simulink model "Powertrain_model_HEV"  (R2021a)
settings: Solver=VariableStepAuto  StartTime=0.0  StopTime=10.0  RelTol=1e-3
values from neighbouring files (symbols this model uses):
  DR = 5.213    [Sim_script.m]    (also in workspace.mat)
  eta_EM_map = [0.5831 0.6831 0.781 0.826 0 0 0 0 0 0.6107 0.7107 0.8049 ... (270 elements, 9x30)]    [workspace.mat]
  MaxLimit = [2.1951    294.39 ... (first row only)    [power_distribute_func.m]
  P_CE_idle = 0    [Sim_script.m]    (also in workspace.mat = 1)
  T_EM_col = [-74.73 -59.49 -53.55 -49.77 -44.93 -40 -34.96 -30.36 -25.1 -20.31 -15.68 -10.18 ... (30 elements, 30x1)]    [workspace.mat]
  T_EM_max = [70 70 70 52 38 28 19 13 9]    [workspace.mat]
  Trans_In = 24.086    [Sim_script.m]    (also in workspace.mat)
  w_CE_idle = 400    [Sim_script.m]    (also in workspace.mat = 32)
  w_EM_row = [0 75 150 225 300 375 450 525 600]    [workspace.mat]
undefined symbols (not defined in the file or in its folder): dailyloadl, eta_EG_map, Res_Torque, T_EG_max, w_EG_row, w_EG_upper
libraries: visionstatistics x1, pid_lib x1
settings Model: Creator=user  LastModifiedBy=user

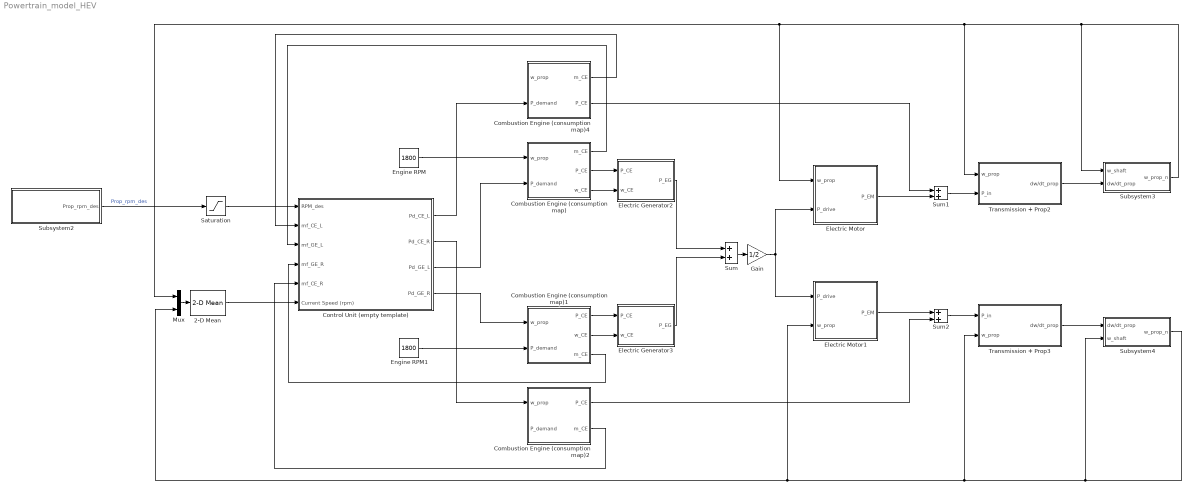
== system Powertrain_model_HEV ==
  2-D Mean : visionstatistics/2-D Mean  run=off  reset_popup=None  directionMode=Entire input  dimension=1  treatSBRowAsCol=on  outputLastDataTypeStr=Inherit: Same as accumulator  accumMode=Binary point scaling  accumWordLength=32  accumFracLength=0  accumLastDataTypeStr=fixdt([],32,0)  roiEnable=off  roiType=Rectangles  roiPortion=Entire ROI  roiOutput=Individual statistics for each ROI  roiFlag=off  roundingMode=Floor  overflowMode=off  accumDataTypeStr=fixdt([],32,0)  outputDataTypeStr=Inherit: Same as accumulator  outputMin=[]  outputMax=[]
      settings: SourceProductBaseCode=VP
  Combustion Engine (consumption map) : Subsystem  Tag=combustion engine  AncestorBlock=|
      | qss_tb_library/Energy Converter/Combustion Engine
      | (consumption map)
  Combustion Engine (consumption map)1 : Subsystem  Tag=combustion engine  AncestorBlock=|
      | qss_tb_library/Energy Converter/Combustion Engine
      | (consumption map)
  Combustion Engine (consumption map)2 : Subsystem  Tag=combustion engine  AncestorBlock=|
      | qss_tb_library/Energy Converter/Combustion Engine
      | (consumption map)
  Combustion Engine (consumption map)4 : Subsystem  Tag=combustion engine  AncestorBlock=|
      | qss_tb_library/Energy Converter/Combustion Engine
      | (consumption map)
  Control Unit (empty template) : Subsystem  Tag=control unit  AncestorBlock=|
      | qss_tb_library/Controller/Control Unit
      | (empty template)
  Electric Generator2 : Subsystem  AncestorBlock=qss_tb_library/Energy Converter/Electric Generator
  Electric Generator3 : Subsystem  AncestorBlock=qss_tb_library/Energy Converter/Electric Generator
  Electric Motor : Subsystem  AncestorBlock=qss_tb_library/Energy Converter/Electric Motor
  Electric Motor1 : Subsystem  AncestorBlock=qss_tb_library/Energy Converter/Electric Motor  mask(Electric Motor){emmapname='qss_em_original_map', scale_EM=1, theta_EM=0.1, P_aux=0}
      mask prompts: emmapname "Motor map name"; scale_EM "Motor scaling factor [-]"; theta_EM "Motor inertia [kg*m2]"; P_aux "Power required by auxiliaries [W]"
      mask help:
      | This block simulates the behaviour of an electric motor. The block is based on an efficiency map. The map is located in the Data/EnergyConvertter/ElectricMotor directory.
      |
      | Input:
      | =====
      | 	w_gear		Speed of the fly wheel [rad/s]
      | 	dw_gear	Acceleration of the fly wheel [rad/s^2]
      | 	T_gear		Torque on the fly wheel [Nm]
      |
      | Output:
      | ======
      | 	P_EM		Power produced by the electric motor [W]
      |
      | Motor map:
      | ======
      | The motor map file must contain the following variables:
      | eta_EM_map		% Efficiency map                [-]
      | w_EM_row		% Motor speed range             [rad/s]
      | T_EM_col		% Motor torque range            [Nm]
      | w_EM_max		% Maximum motor speed           [rad/s]
      | load T_EM_max	% Maximum motor torque          [Nm]
      mask init:
      | init_EM;
  Engine RPM : Constant  Value=1800
  Engine RPM1 : Constant  Value=1800
  Gain : Gain  Gain=1/2
  Mux : Mux  Inputs=2
  Saturation : Saturate  UpperLimit=inf  LowerLimit=w_CE_idle
  Subsystem2 : Subsystem  TreatAsAtomicUnit=on
  Subsystem3 : Subsystem
  Subsystem4 : Subsystem
  Sum : Sum
  Sum1 : Sum
  Sum2 : Sum
  Transmission + Prop2 : Subsystem
  Transmission + Prop3 : Subsystem
  wires:
  Combustion Engine (consumption map)1/1(P_CE) -> Electric Generator3/1(P_CE)
  Engine RPM/1 -> Combustion Engine (consumption map)/1(w_prop)
  Combustion Engine (consumption map)/2(P_CE) -> Electric Generator2/1(P_CE)
  Transmission + Prop2/1(dw/dt_prop) -> Subsystem3/2(dw/dt_prop)
  Transmission + Prop3/1(dw/dt_prop) -> Subsystem4/1(dw/dt_prop)
  Subsystem3/1(w_prop_n) -> Subsystem3/1(w_shaft), Transmission + Prop2/1(w_prop), Electric Motor/1(w_prop), Mux/1
  Electric Motor1/1(P_EM) -> Sum2/1
  Combustion Engine (consumption map)1/2(w_CE) -> Electric Generator3/2(w_CE)
  Subsystem4/1(w_prop_n) -> Subsystem4/2(w_shaft), Transmission + Prop3/2(w_prop), Mux/2, Electric Motor1/2(w_prop)
  Electric Generator3/1(P_EG) -> Sum/2
  Sum2/1 -> Transmission + Prop3/1(P_in)
  Combustion Engine (consumption map)4/2(P_CE) -> Sum1/1
  Sum1/1 -> Transmission + Prop2/2(P_in)
  Gain/1 -> Electric Motor/2(P_drive), Electric Motor1/1(P_drive)
  Combustion Engine (consumption map)/1(m_CE) -> Control Unit (empty template)/3(mf_GE_L)
  Electric Motor/1(P_EM) -> Sum1/2
  Control Unit (empty template)/4(Pd_GE_R) -> Combustion Engine (consumption map)1/1(w_prop)
  Combustion Engine (consumption map)/3(w_CE) -> Electric Generator2/2(w_CE)
  Combustion Engine (consumption map)2/2(m_CE) -> Control Unit (empty template)/5(mf_CE_R)
  Combustion Engine (consumption map)4/1(m_CE) -> Control Unit (empty template)/2(mf_CE_L)
  Engine RPM1/1 -> Combustion Engine (consumption map)1/2(P_demand)
  Electric Generator2/1(P_EG) -> Sum/1
  Mux/1 -> 2-D Mean/1
  Control Unit (empty template)/3(Pd_GE_L) -> Combustion Engine (consumption map)/2(P_demand)
  Control Unit (empty template)/2(Pd_CE_R) -> Combustion Engine (consumption map)2/1(w_prop)
  Sum/1 -> Gain/1
  Control Unit (empty template)/1(Pd_CE_L) -> Combustion Engine (consumption map)4/2(P_demand)
  2-D Mean/1 -> Control Unit (empty template)/6(Current Speed (rpm))
  Combustion Engine (consumption map)1/3(m_CE) -> Control Unit (empty template)/4(mf_GE_R)
  Combustion Engine (consumption map)2/1(P_CE) -> Sum2/2
  Subsystem2/1(Prop_rpm_des) -> Saturation/1  "Prop_rpm_des"
  Saturation/1 -> Control Unit (empty template)/1(RPM_des)

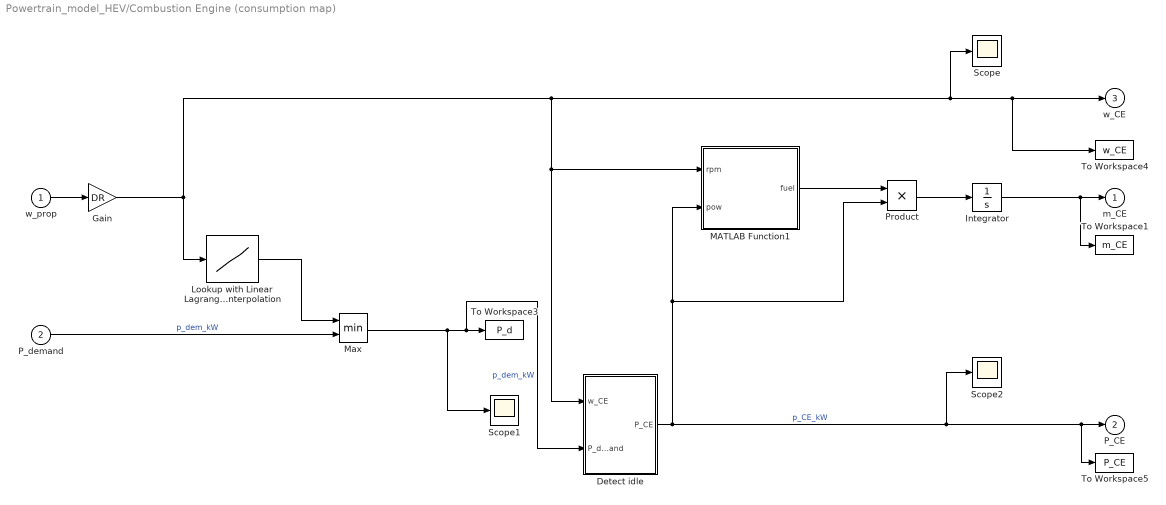
== system Powertrain_model_HEV/Combustion Engine (consumption map) ==
  w_prop : Inport
  P_demand : Inport  Port=2
  Detect idle : Subsystem
  Gain : Gain  Gain=DR
  Integrator : Integrator
  Lookup with Linear Lagrange Interpolation : Lookup_n-D  NumberOfTableDimensions=1  BreakpointsForDimension1=MaxLimit.('RPM')  Table=MaxLimit.('Pow_kW_')  InterpMethod=Linear Lagrange  InternalRulePriority=Speed  RndMeth=Simplest  InputSameDT=on
  MATLAB Function1 : MATLAB Function  TreatAsAtomicUnit=on
  Max : MinMax  Inputs=2
  Product : Product
  Scope : Scope
  Scope1 : Scope
  Scope2 : Scope
  To Workspace1 : ToWorkspace  VariableName=m_CE  SampleTime=-1
      settings: Save2DSignal=2-D array (concatenate along first dimension)
  To Workspace3 : ToWorkspace  VariableName=P_d  SampleTime=-1
      settings: Save2DSignal=2-D array (concatenate along first dimension)
  To Workspace4 : ToWorkspace  VariableName=w_CE  SampleTime=-1
      settings: Save2DSignal=2-D array (concatenate along first dimension)
  To Workspace5 : ToWorkspace  VariableName=P_CE  SampleTime=-1
      settings: Save2DSignal=2-D array (concatenate along first dimension)
  m_CE : Outport  InitialOutput=0
  P_CE : Outport  Port=2  InitialOutput=0
  w_CE : Outport  Port=3  InitialOutput=0
  wires:
  Integrator/1 -> To Workspace1/1, m_CE/1
  w_prop/1 -> Gain/1
  Detect idle/1(P_CE) -> Scope2/1, To Workspace5/1, P_CE/1, Product/2, MATLAB Function1/2(pow)  "p_CE_kW"
  Lookup with Linear Lagrange Interpolation/1 -> Max/1
  MATLAB Function1/1(fuel) -> Product/1
  Gain/1 -> w_CE/1, To Workspace4/1, Scope/1, Detect idle/1(w_CE), MATLAB Function1/1(rpm), Lookup with Linear Lagrange Interpolation/1
  Product/1 -> Integrator/1
  Max/1 -> Scope1/1, Detect idle/2(P_demand), To Workspace3/1  "p_dem_kW"
  P_demand/1 -> Max/2  "p_dem_kW"

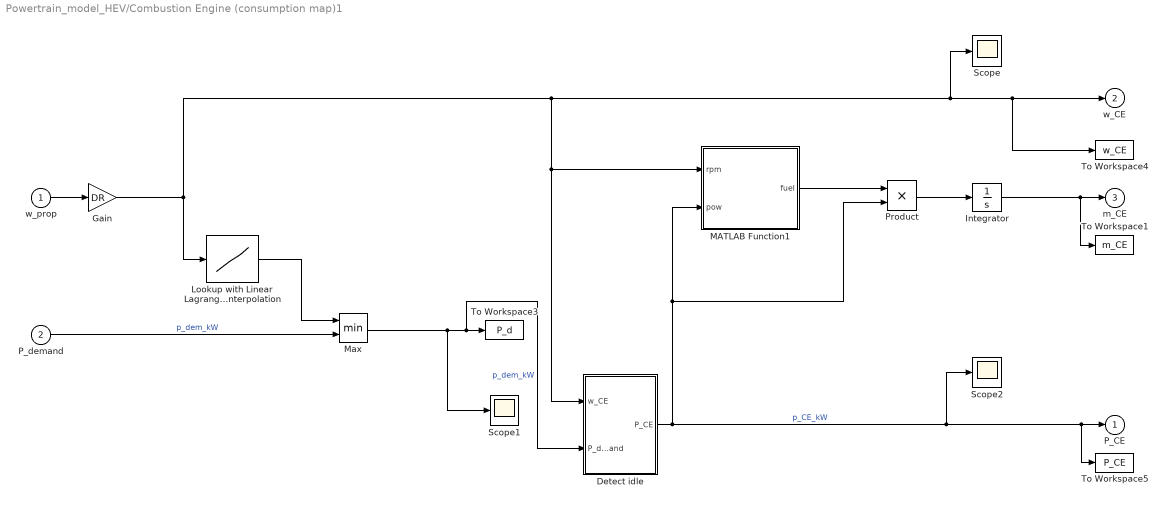
== system Powertrain_model_HEV/Combustion Engine (consumption map)1 ==
  w_prop : Inport
  P_demand : Inport  Port=2
  Detect idle : Subsystem
  Gain : Gain  Gain=DR
  Integrator : Integrator
  Lookup with Linear Lagrange Interpolation : Lookup_n-D  NumberOfTableDimensions=1  BreakpointsForDimension1=MaxLimit.('RPM')  Table=MaxLimit.('Pow_kW_')  InterpMethod=Linear Lagrange  InternalRulePriority=Speed  RndMeth=Simplest  InputSameDT=on
  MATLAB Function1 : MATLAB Function  TreatAsAtomicUnit=on
  Max : MinMax  Inputs=2
  Product : Product
  Scope : Scope
  Scope1 : Scope
  Scope2 : Scope
  To Workspace1 : ToWorkspace  VariableName=m_CE  SampleTime=-1
      settings: Save2DSignal=2-D array (concatenate along first dimension)
  To Workspace3 : ToWorkspace  VariableName=P_d  SampleTime=-1
      settings: Save2DSignal=2-D array (concatenate along first dimension)
  To Workspace4 : ToWorkspace  VariableName=w_CE  SampleTime=-1
      settings: Save2DSignal=2-D array (concatenate along first dimension)
  To Workspace5 : ToWorkspace  VariableName=P_CE  SampleTime=-1
      settings: Save2DSignal=2-D array (concatenate along first dimension)
  P_CE : Outport  InitialOutput=0
  w_CE : Outport  Port=2  InitialOutput=0
  m_CE : Outport  Port=3  InitialOutput=0
  wires:
  Integrator/1 -> To Workspace1/1, m_CE/1
  w_prop/1 -> Gain/1
  Detect idle/1(P_CE) -> Scope2/1, To Workspace5/1, P_CE/1, Product/2, MATLAB Function1/2(pow)  "p_CE_kW"
  Lookup with Linear Lagrange Interpolation/1 -> Max/1
  MATLAB Function1/1(fuel) -> Product/1
  Gain/1 -> w_CE/1, To Workspace4/1, Scope/1, Detect idle/1(w_CE), MATLAB Function1/1(rpm), Lookup with Linear Lagrange Interpolation/1
  Product/1 -> Integrator/1
  Max/1 -> Scope1/1, Detect idle/2(P_demand), To Workspace3/1  "p_dem_kW"
  P_demand/1 -> Max/2  "p_dem_kW"

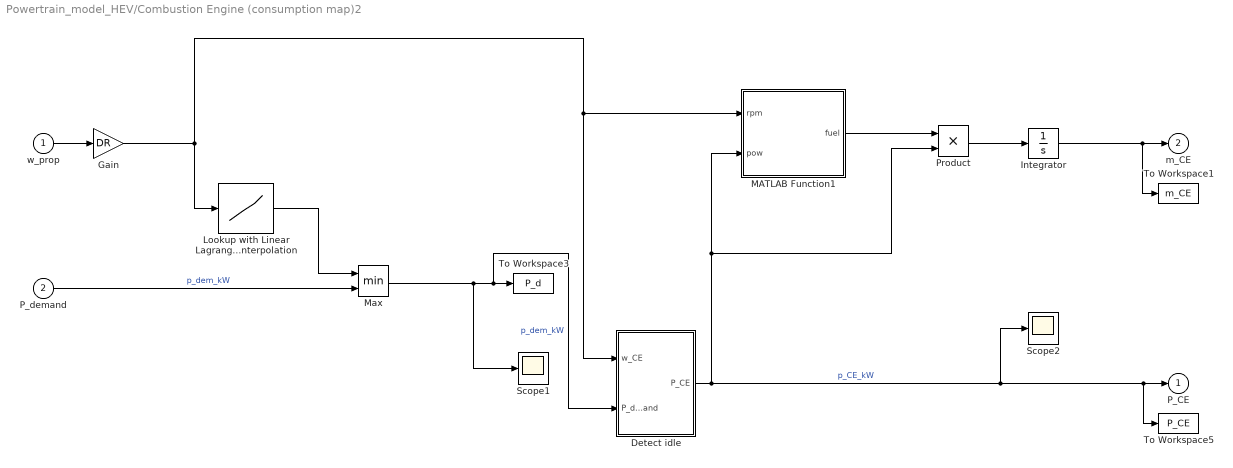
== system Powertrain_model_HEV/Combustion Engine (consumption map)2 ==
  w_prop : Inport
  P_demand : Inport  Port=2
  Detect idle : Subsystem
  Gain : Gain  Gain=DR
  Integrator : Integrator
  Lookup with Linear Lagrange Interpolation : Lookup_n-D  NumberOfTableDimensions=1  BreakpointsForDimension1=MaxLimit.('RPM')  Table=MaxLimit.('Pow_kW_')  InterpMethod=Linear Lagrange  InternalRulePriority=Speed  RndMeth=Simplest  InputSameDT=on
  MATLAB Function1 : MATLAB Function  TreatAsAtomicUnit=on
  Max : MinMax  Inputs=2
  Product : Product
  Scope1 : Scope
  Scope2 : Scope
  To Workspace1 : ToWorkspace  VariableName=m_CE  SampleTime=-1
      settings: Save2DSignal=2-D array (concatenate along first dimension)
  To Workspace3 : ToWorkspace  VariableName=P_d  SampleTime=-1
      settings: Save2DSignal=2-D array (concatenate along first dimension)
  To Workspace5 : ToWorkspace  VariableName=P_CE  SampleTime=-1
      settings: Save2DSignal=2-D array (concatenate along first dimension)
  P_CE : Outport  InitialOutput=0
  m_CE : Outport  Port=2  InitialOutput=0
  wires:
  Integrator/1 -> To Workspace1/1, m_CE/1
  w_prop/1 -> Gain/1
  Detect idle/1(P_CE) -> Scope2/1, To Workspace5/1, P_CE/1, Product/2, MATLAB Function1/2(pow)  "p_CE_kW"
  Lookup with Linear Lagrange Interpolation/1 -> Max/1
  MATLAB Function1/1(fuel) -> Product/1
  Gain/1 -> Detect idle/1(w_CE), MATLAB Function1/1(rpm), Lookup with Linear Lagrange Interpolation/1
  Product/1 -> Integrator/1
  Max/1 -> Scope1/1, Detect idle/2(P_demand), To Workspace3/1  "p_dem_kW"
  P_demand/1 -> Max/2  "p_dem_kW"

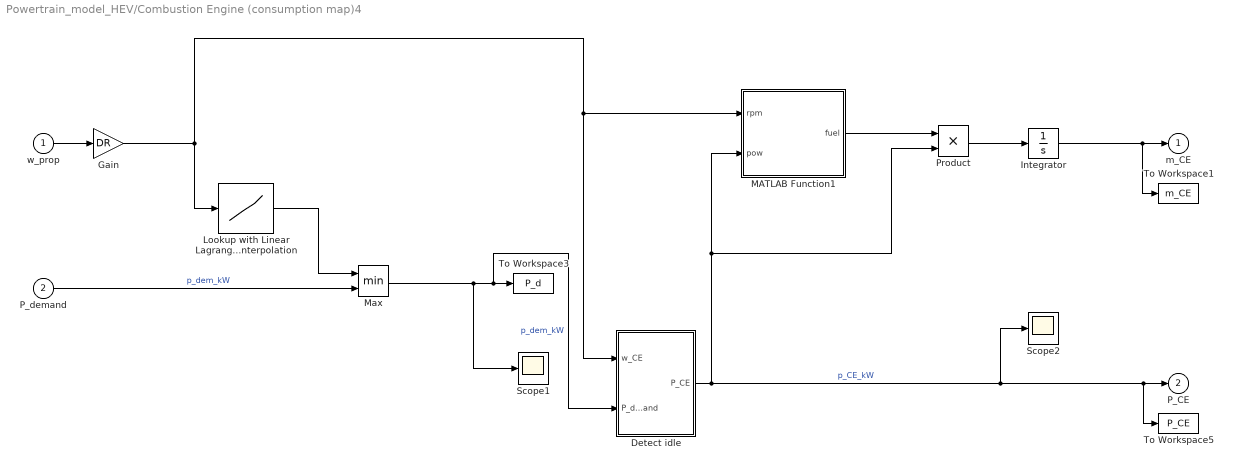
== system Powertrain_model_HEV/Combustion Engine (consumption map)4 ==
  w_prop : Inport
  P_demand : Inport  Port=2
  Detect idle : Subsystem
  Gain : Gain  Gain=DR
  Integrator : Integrator
  Lookup with Linear Lagrange Interpolation : Lookup_n-D  NumberOfTableDimensions=1  BreakpointsForDimension1=MaxLimit.('RPM')  Table=MaxLimit.('Pow_kW_')  InterpMethod=Linear Lagrange  InternalRulePriority=Speed  RndMeth=Simplest  InputSameDT=on
  MATLAB Function1 : MATLAB Function  TreatAsAtomicUnit=on
  Max : MinMax  Inputs=2
  Product : Product
  Scope1 : Scope
  Scope2 : Scope
  To Workspace1 : ToWorkspace  VariableName=m_CE  SampleTime=-1
      settings: Save2DSignal=2-D array (concatenate along first dimension)
  To Workspace3 : ToWorkspace  VariableName=P_d  SampleTime=-1
      settings: Save2DSignal=2-D array (concatenate along first dimension)
  To Workspace5 : ToWorkspace  VariableName=P_CE  SampleTime=-1
      settings: Save2DSignal=2-D array (concatenate along first dimension)
  m_CE : Outport  InitialOutput=0
  P_CE : Outport  Port=2  InitialOutput=0
  wires:
  Integrator/1 -> To Workspace1/1, m_CE/1
  w_prop/1 -> Gain/1
  Detect idle/1(P_CE) -> Scope2/1, To Workspace5/1, P_CE/1, Product/2, MATLAB Function1/2(pow)  "p_CE_kW"
  Lookup with Linear Lagrange Interpolation/1 -> Max/1
  MATLAB Function1/1(fuel) -> Product/1
  Gain/1 -> Detect idle/1(w_CE), MATLAB Function1/1(rpm), Lookup with Linear Lagrange Interpolation/1
  Product/1 -> Integrator/1
  Max/1 -> Scope1/1, Detect idle/2(P_demand), To Workspace3/1  "p_dem_kW"
  P_demand/1 -> Max/2  "p_dem_kW"

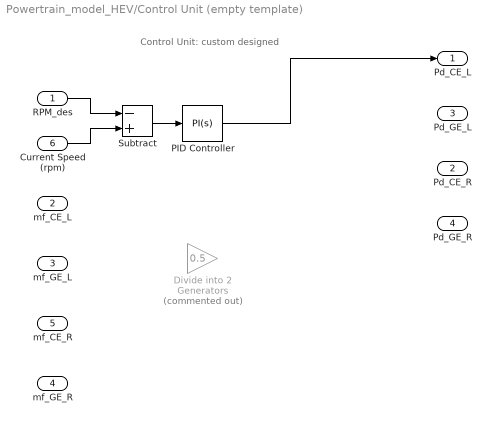
== system Powertrain_model_HEV/Control Unit (empty template) ==
  note: Control Unit: custom designed
  RPM_des : Inport
  mf_CE_L : Inport  Port=2
  mf_GE_L : Inport  Port=3
  mf_GE_R : Inport  Port=4
  mf_CE_R : Inport  Port=5
  Current Speed (rpm) : Inport  Port=6
  Divide into 2 Generators : Gain  Commented=on  Gain=0.5
  PID Controller : pid_lib/PID Controller  Controller=PI  Form=Parallel  TimeDomain=Continuous-time  UseExternalTs=off  SampleTime=-1  IntegratorMethod=Forward Euler  FilterMethod=Forward Euler  ControllerParametersSource=internal  P=4  I=1.2  D=0  UseFilter=on  N=100  TunerSelectOption=Transfer Function Based (PID Tuner App)  InitialConditionSource=internal  InitialConditionForIntegrator=0  InitialConditionForFilter=0  DifferentiatorICPrevScaledInput=0  ExternalReset=none  TrackingMode=off  Kt=1  LimitOutput=off  SatLimitsSource=internal  UpperSaturationLimit=inf  LowerSaturationLimit=-inf  LinearizeAsGain=on  AntiWindupMode=none  Kb=1  POutMin=[]  POutMax=[]  IOutMin=[]  IOutMax=[]  DOutMin=[]  DOutMax=[]  NOutMin=[]  NOutMax=[]  SumOutMin=[]  SumOutMax=[]  SaturationOutMin=[]  SaturationOutMax=[]  PParamMin=[]  PParamMax=[]  IParamMin=[]  IParamMax=[]  DParamMin=[]  DParamMax=[]  NParamMin=[]  NParamMax=[]  KbParamMin=[]  KbParamMax=[]  KtParamMin=[]  KtParamMax=[]  KbOutMin=[]  KbOutMax=[]  KtOutMin=[]  KtOutMax=[]  IntegratorOutMin=[]  IntegratorOutMax=[]  FilterOutMin=[]  FilterOutMax=[]  SumI1OutMin=[]  SumI1OutMax=[]  SumI2OutMin=[]  SumI2OutMax=[]  SumI3OutMin=[]  SumI3OutMax=[]  SumI4OutMin=[]  SumI4OutMax=[]  SumDOutMin=[]  SumDOutMax=[]  DifferentiatorOutMin=[]  DifferentiatorOutMax=[]  FilterDiffOutCoefMin=[]  FilterDiffOutCoefMax=[]  ReciprocalOutMin=[]  ReciprocalOutMax=[]  SumDenOutMin=[]  SumDenOutMax=[]  SumNumOutMin=[]  SumNumOutMax=[]  DivideOutMin=[]  DivideOutMax=[]  UdiffTsProdOutMin=[]  UdiffTsProdOutMax=[]  NTsProdOutMin=[]  NTsProdOutMax=[]  UintegralTsProdOutMin=[]  UintegralTsProdOutMax=[]  UngainTsProdOutMin=[]  UngainTsProdOutMax=[]  IntegratorContinuousStateAttributes=''  IntegratorStateMustResolveToSignalObject=off  IntegratorRTWStateStorageClass=Auto  FilterContinuousStateAttributes=''  FilterStateMustResolveToSignalObject=off  FilterRTWStateStorageClass=Auto  ParallelPVariant=InternalParameters  IdealPVariant=Disabled  IVariant=InternalParameters  DVariant=Disabled  IntegratorVariant=Continuous  SatVariant=Disabled  AWVariant=Passthrough  PCopyVariant=Disabled  TRVariant=Disabled  FdbkBlocksVariant=Forward  IdealPFdbkVariant=Disabled  SatFdbkVariant=Disabled  DerivativeFilterVariant=Disabled  NVariant=Disabled  NCopyVariant=Disabled_SignalSpec  FilterICVariant=Disabled  IntegratorICVariant=InternalICs  ExternalResetVariant=Disabled  TRSumVariant=Passthrough  SumFdbkVariant=Disabled  SumVariant=Sum_PI  TsampFilterVariant=InternalTs  TsampNgainVariant=Passthrough  TsampIntegralVariant=Passthrough  ExternalSaturationOutDataTypeStr=Inherit: Same as second input
  Subtract : Sum  Inputs=-+
  Pd_CE_L : Outport  InitialOutput=0
  Pd_CE_R : Outport  Port=2  InitialOutput=0
  Pd_GE_L : Outport  Port=3  InitialOutput=0
  Pd_GE_R : Outport  Port=4  InitialOutput=0
  wires:
  Current Speed (rpm)/1 -> Subtract/2
  RPM_des/1 -> Subtract/1
  PID Controller/1 -> Pd_CE_L/1
  Subtract/1 -> PID Controller/1

== system Powertrain_model_HEV/Electric Generator2 ==
  P_CE : Inport
  w_CE : Inport  Port=2
  Detect overload and overspeed : Subsystem
  Divide : Product  Inputs=/*
  "Efficiency eta = f(w, T)" : Lookup2D  RowIndex=w_EG_row  ColumnIndex=T_EG_col  Table=eta_EG_map
  Product : Product  Inputs=3  InputSameDT=on  RndMeth=Zero  SaturateOnIntegerOverflow=on  OutDataTypeStr=Inherit: Same as first input
  To Workspace1 : ToWorkspace  VariableName=w_EG  SampleTime=-1
  To Workspace2 : ToWorkspace  VariableName=T_EG  SampleTime=-1
  To Workspace5 : ToWorkspace  VariableName=P_EG  SampleTime=-1
  P_EG : Outport  InitialOutput=0
  wires:
  Product/1 -> To Workspace5/1, P_EG/1
  "Efficiency eta = f(w, T)"/1 -> Product/1
  Divide/1 -> To Workspace2/1, Detect overload and overspeed/2(T_EG), "Efficiency eta = f(w, T)"/2, Product/2
  P_CE/1 -> Divide/2
  w_CE/1 -> To Workspace1/1, Detect overload and overspeed/1(w_EG), "Efficiency eta = f(w, T)"/1, Product/3, Divide/1

== system Powertrain_model_HEV/Electric Generator3 ==
  P_CE : Inport
  w_CE : Inport  Port=2
  Detect overload and overspeed : Subsystem
  Divide : Product  Inputs=/*
  "Efficiency eta = f(w, T)" : Lookup2D  RowIndex=w_EG_row  ColumnIndex=T_EG_col  Table=eta_EG_map
  Product : Product  Inputs=3  InputSameDT=on  RndMeth=Zero  SaturateOnIntegerOverflow=on  OutDataTypeStr=Inherit: Same as first input
  To Workspace1 : ToWorkspace  VariableName=w_EG  SampleTime=-1
  To Workspace2 : ToWorkspace  VariableName=T_EG  SampleTime=-1
  To Workspace5 : ToWorkspace  VariableName=P_EG  SampleTime=-1
  P_EG : Outport  InitialOutput=0
  wires:
  Product/1 -> To Workspace5/1, P_EG/1
  "Efficiency eta = f(w, T)"/1 -> Product/1
  Divide/1 -> To Workspace2/1, Detect overload and overspeed/2(T_EG), "Efficiency eta = f(w, T)"/2, Product/2
  P_CE/1 -> Divide/2
  w_CE/1 -> To Workspace1/1, Detect overload and overspeed/1(w_EG), "Efficiency eta = f(w, T)"/1, Product/3, Divide/1

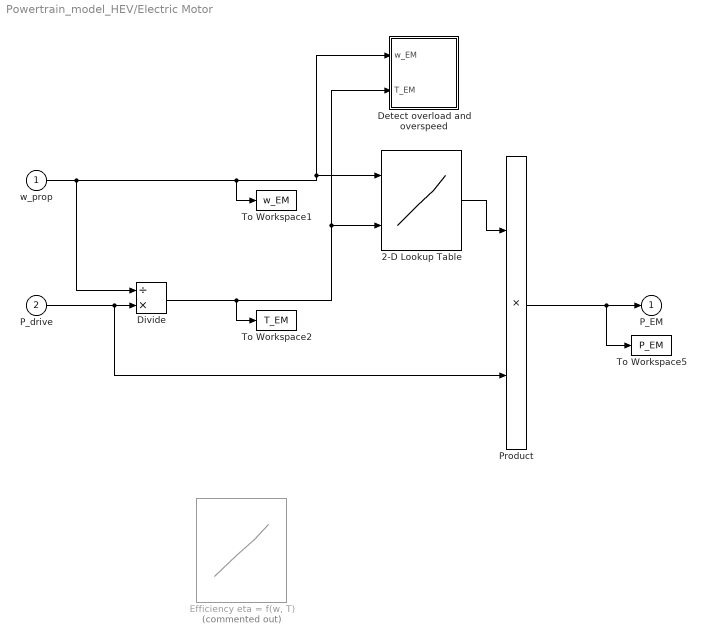
== system Powertrain_model_HEV/Electric Motor ==
  w_prop : Inport
  P_drive : Inport  Port=2
  2-D Lookup Table : Lookup_n-D  BreakpointsForDimension1=w_EM_row  BreakpointsForDimension2=T_EM_col  Table=eta_EM_map  InterpMethod=Cubic spline  ExtrapMethod=Cubic spline  InternalRulePriority=Speed  RndMeth=Simplest  InputSameDT=on
      settings: InputPortMap=u0,u1
  Detect overload and overspeed : Subsystem
  Divide : Product  Inputs=/*
  "Efficiency eta = f(w, T)" : Lookup2D  Commented=on  RowIndex=w_EM_row  ColumnIndex=T_EM_col  Table=eta_EM_map
  Product : Product  InputSameDT=on  RndMeth=Zero  SaturateOnIntegerOverflow=on  OutDataTypeStr=Inherit: Same as first input
  To Workspace1 : ToWorkspace  VariableName=w_EM  SampleTime=-1
  To Workspace2 : ToWorkspace  VariableName=T_EM  SampleTime=-1
  To Workspace5 : ToWorkspace  VariableName=P_EM  SampleTime=-1
  P_EM : Outport  InitialOutput=0
  wires:
  Product/1 -> To Workspace5/1, P_EM/1
  Divide/1 -> To Workspace2/1, 2-D Lookup Table/2, Detect overload and overspeed/2(T_EM)
  P_drive/1 -> Product/2, Divide/2
  2-D Lookup Table/1 -> Product/1
  w_prop/1 -> Divide/1, To Workspace1/1, 2-D Lookup Table/1, Detect overload and overspeed/1(w_EM)

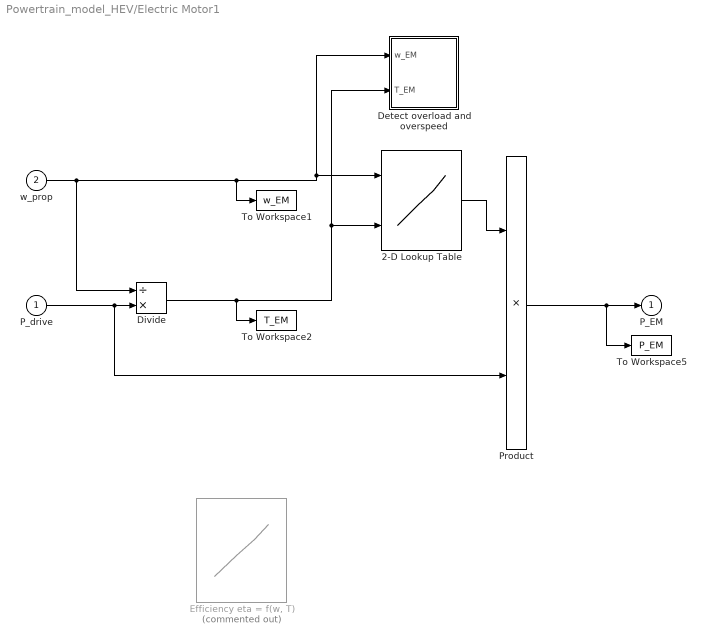
== system Powertrain_model_HEV/Electric Motor1 ==
  P_drive : Inport
  w_prop : Inport  Port=2
  2-D Lookup Table : Lookup_n-D  BreakpointsForDimension1=w_EM_row  BreakpointsForDimension2=T_EM_col  Table=eta_EM_map  InterpMethod=Cubic spline  ExtrapMethod=Cubic spline  InternalRulePriority=Speed  RndMeth=Simplest  InputSameDT=on
      settings: InputPortMap=u0,u1
  Detect overload and overspeed : Subsystem
  Divide : Product  Inputs=/*
  "Efficiency eta = f(w, T)" : Lookup2D  Commented=on  RowIndex=w_EM_row  ColumnIndex=T_EM_col  Table=eta_EM_map
  Product : Product  InputSameDT=on  RndMeth=Zero  SaturateOnIntegerOverflow=on  OutDataTypeStr=Inherit: Same as first input
  To Workspace1 : ToWorkspace  VariableName=w_EM  SampleTime=-1
  To Workspace2 : ToWorkspace  VariableName=T_EM  SampleTime=-1
  To Workspace5 : ToWorkspace  VariableName=P_EM  SampleTime=-1
  P_EM : Outport  InitialOutput=0
  wires:
  w_prop/1 -> Detect overload and overspeed/1(w_EM), 2-D Lookup Table/1, To Workspace1/1, Divide/1
  2-D Lookup Table/1 -> Product/1
  P_drive/1 -> Divide/2, Product/2
  Divide/1 -> Detect overload and overspeed/2(T_EM), 2-D Lookup Table/2, To Workspace2/1
  Product/1 -> P_EM/1, To Workspace5/1

== system Powertrain_model_HEV/Subsystem2 ==
  1-D Lookup Table : Lookup_n-D  NumberOfTableDimensions=1  BreakpointsForDimension1=[1:10800]  Table=dailyloadl.('m_sec')  InternalRulePriority=Speed  RndMeth=Simplest  InputSameDT=on
  Clock : Clock
  To Workspace3 : ToWorkspace  VariableName=t  SampleTime=-1
      settings: Save2DSignal=2-D array (concatenate along first dimension)
  To Workspace4 : ToWorkspace  VariableName=rpm_des  SampleTime=-1
      settings: Save2DSignal=2-D array (concatenate along first dimension)
  Prop_rpm_des : Outport
  wires:
  Clock/1 -> To Workspace3/1, 1-D Lookup Table/1
  1-D Lookup Table/1 -> Prop_rpm_des/1, To Workspace4/1

== system Powertrain_model_HEV/Subsystem3 ==
  w_shaft : Inport
  dw/dt_prop : Inport  Port=2
  Add : Sum
  Gain : Gain  Gain=1/9.5493
  Gain1 : Gain  Gain=1/DR
  Integrator : Integrator  InitialCondition=w_CE_idle
  Saturation : Saturate  UpperLimit=inf  LowerLimit=w_CE_idle
  w_prop_n : Outport
  wires:
  dw/dt_prop/1 -> Integrator/1
  Integrator/1 -> Gain/1
  Saturation/1 -> w_prop_n/1
  Gain/1 -> Add/2
  w_shaft/1 -> Gain1/1
  Gain1/1 -> Add/1
  Add/1 -> Saturation/1

== system Powertrain_model_HEV/Subsystem4 ==
  dw/dt_prop : Inport
  w_shaft : Inport  Port=2
  Add : Sum
  Gain : Gain  Gain=1/9.5493
  Gain1 : Gain  Gain=1/DR
  Integrator : Integrator  InitialCondition=w_CE_idle
  Saturation : Saturate  UpperLimit=inf  LowerLimit=w_CE_idle
  w_prop_n : Outport
  wires:
  dw/dt_prop/1 -> Integrator/1
  Integrator/1 -> Gain/1
  Saturation/1 -> w_prop_n/1
  Gain/1 -> Add/2
  w_shaft/1 -> Gain1/1
  Gain1/1 -> Add/1
  Add/1 -> Saturation/1

== system Powertrain_model_HEV/Transmission + Prop2 ==
  w_prop : Inport
  P_in : Inport  Port=2
  Divide : Product  Inputs=*/
  Drive Ratio : Gain  Gain=DR
  Gain : Gain  Gain=DR
  Gain2 : Gain  Gain=9.5488*1000
  Gearbox+Prop Inertia : Gain  Gain=1/Trans_In
  Lookup with Linear Point-slope Interpolation : Lookup_n-D  NumberOfTableDimensions=1  BreakpointsForDimension1=Res_Torque.('RPMEngine')  Table=Res_Torque.('TorqueNM')  InternalRulePriority=Speed  RndMeth=Simplest  InputSameDT=on
  Scope : Scope
  Subtract : Sum  Inputs=+-
  dw/dt_prop : Outport
  wires:
  Lookup with Linear Point-slope Interpolation/1 -> Subtract/2  "T_res"
  P_in/1 -> Divide/1
  Subtract/1 -> Scope/1, Drive Ratio/1
  Gearbox+Prop Inertia/1 -> dw/dt_prop/1  "dw/dt_prop"
  Drive Ratio/1 -> Gearbox+Prop Inertia/1
  Divide/1 -> Gain2/1  "T_CE"
  Gain/1 -> Divide/2, Lookup with Linear Point-slope Interpolation/1
  Gain2/1 -> Subtract/1
  w_prop/1 -> Gain/1  "prop_rads"

== system Powertrain_model_HEV/Transmission + Prop3 ==
  P_in : Inport
  w_prop : Inport  Port=2
  Divide : Product  Inputs=*/
  Drive Ratio : Gain  Gain=DR
  Gain : Gain  Gain=DR
  Gain2 : Gain  Gain=9.5488*1000
  Gearbox+Prop Inertia : Gain  Gain=1/Trans_In
  Lookup with Linear Point-slope Interpolation : Lookup_n-D  NumberOfTableDimensions=1  BreakpointsForDimension1=Res_Torque.('RPMEngine')  Table=Res_Torque.('TorqueNM')  InternalRulePriority=Speed  RndMeth=Simplest  InputSameDT=on
  Scope : Scope
  Subtract : Sum  Inputs=+-
  dw/dt_prop : Outport
  wires:
  Lookup with Linear Point-slope Interpolation/1 -> Subtract/2  "T_res"
  P_in/1 -> Divide/1
  Subtract/1 -> Scope/1, Drive Ratio/1
  Gearbox+Prop Inertia/1 -> dw/dt_prop/1  "dw/dt_prop"
  Drive Ratio/1 -> Gearbox+Prop Inertia/1
  Divide/1 -> Gain2/1  "T_CE"
  Gain/1 -> Divide/2, Lookup with Linear Point-slope Interpolation/1
  Gain2/1 -> Subtract/1
  w_prop/1 -> Gain/1  "prop_rads"

== system Powertrain_model_HEV/Combustion Engine (consumption map)/Detect idle ==
  w_CE : Inport
  P_demand : Inport  Port=2
  Constant3 : Constant  Value=P_CE_idle
  Idle detection : Fcn  Expr=(u(1) <= w_CE_idle) * (u(2) <= P_CE_idle)
  Mux : Mux  Inputs=2
  P_demand1 : InportShadow  Port=2
  Switch2 : Switch  Threshold=0.5  SaturateOnIntegerOverflow=on  InputSameDT=on
  P_CE : Outport  InitialOutput=0
  wires:
  Constant3/1 -> Switch2/1
  Switch2/1 -> P_CE/1
  P_demand1/1 -> Switch2/3
  Idle detection/1 -> Switch2/2
  w_CE/1 -> Mux/1
  P_demand/1 -> Mux/2
  Mux/1 -> Idle detection/1

== system Powertrain_model_HEV/Combustion Engine (consumption map)1/Detect idle ==
  w_CE : Inport
  P_demand : Inport  Port=2
  Constant3 : Constant  Value=P_CE_idle
  Idle detection : Fcn  Expr=(u(1) <= w_CE_idle) * (u(2) <= P_CE_idle)
  Mux : Mux  Inputs=2
  P_demand1 : InportShadow  Port=2
  Switch2 : Switch  Threshold=0.5  SaturateOnIntegerOverflow=on  InputSameDT=on
  P_CE : Outport  InitialOutput=0
  wires:
  Constant3/1 -> Switch2/1
  Switch2/1 -> P_CE/1
  P_demand1/1 -> Switch2/3
  Idle detection/1 -> Switch2/2
  w_CE/1 -> Mux/1
  P_demand/1 -> Mux/2
  Mux/1 -> Idle detection/1

== system Powertrain_model_HEV/Combustion Engine (consumption map)2/Detect idle ==
  w_CE : Inport
  P_demand : Inport  Port=2
  Constant3 : Constant  Value=P_CE_idle
  Idle detection : Fcn  Expr=(u(1) <= w_CE_idle) * (u(2) <= P_CE_idle)
  Mux : Mux  Inputs=2
  P_demand1 : InportShadow  Port=2
  Switch2 : Switch  Threshold=0.5  SaturateOnIntegerOverflow=on  InputSameDT=on
  P_CE : Outport  InitialOutput=0
  wires:
  Constant3/1 -> Switch2/1
  Switch2/1 -> P_CE/1
  P_demand1/1 -> Switch2/3
  Idle detection/1 -> Switch2/2
  w_CE/1 -> Mux/1
  P_demand/1 -> Mux/2
  Mux/1 -> Idle detection/1

== system Powertrain_model_HEV/Combustion Engine (consumption map)4/Detect idle ==
  w_CE : Inport
  P_demand : Inport  Port=2
  Constant3 : Constant  Value=P_CE_idle
  Idle detection : Fcn  Expr=(u(1) <= w_CE_idle) * (u(2) <= P_CE_idle)
  Mux : Mux  Inputs=2
  P_demand1 : InportShadow  Port=2
  Switch2 : Switch  Threshold=0.5  SaturateOnIntegerOverflow=on  InputSameDT=on
  P_CE : Outport  InitialOutput=0
  wires:
  Constant3/1 -> Switch2/1
  Switch2/1 -> P_CE/1
  P_demand1/1 -> Switch2/3
  Idle detection/1 -> Switch2/2
  w_CE/1 -> Mux/1
  P_demand/1 -> Mux/2
  Mux/1 -> Idle detection/1

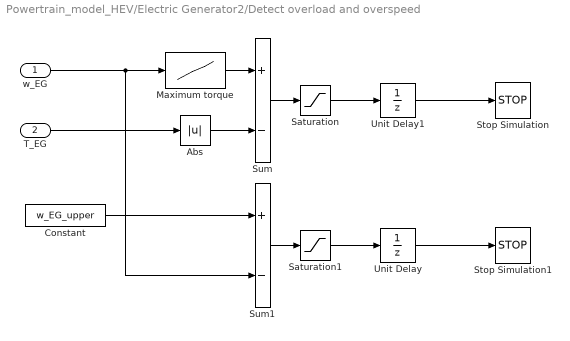
== system Powertrain_model_HEV/Electric Generator2/Detect overload and overspeed ==
  w_EG : Inport
  T_EG : Inport  Port=2
  Abs : Abs  SaturateOnIntegerOverflow=on
  Constant : Constant  Value=w_EG_upper
  Maximum torque : Lookup  InputValues=w_EG_row  Table=T_EG_max  SaturateOnIntegerOverflow=on
  Saturation : Saturate  UpperLimit=0  LowerLimit=-inf
  Saturation1 : Saturate  UpperLimit=0  LowerLimit=-inf
  Stop Simulation : Stop
  Stop Simulation1 : Stop
  Sum : Sum  Inputs=+-  InputSameDT=on  SaturateOnIntegerOverflow=on  OutDataTypeStr=Inherit: Same as first input
  Sum1 : Sum  Inputs=+-  InputSameDT=on  SaturateOnIntegerOverflow=on  OutDataTypeStr=Inherit: Same as first input
  Unit Delay : UnitDelay  SampleTime=-1  HasFrameUpgradeWarning=on
  Unit Delay1 : UnitDelay  SampleTime=-1  HasFrameUpgradeWarning=on
  wires:
  Unit Delay1/1 -> Stop Simulation/1
  Unit Delay/1 -> Stop Simulation1/1
  Saturation1/1 -> Unit Delay/1
  Sum1/1 -> Saturation1/1
  Constant/1 -> Sum1/1
  Saturation/1 -> Unit Delay1/1
  Abs/1 -> Sum/2
  Maximum torque/1 -> Sum/1
  T_EG/1 -> Abs/1
  w_EG/1 -> Sum1/2, Maximum torque/1
  Sum/1 -> Saturation/1

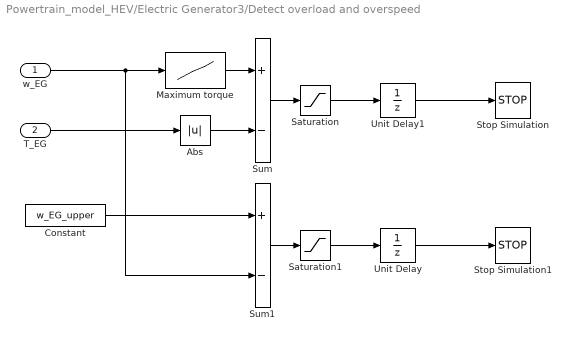
== system Powertrain_model_HEV/Electric Generator3/Detect overload and overspeed ==
  w_EG : Inport
  T_EG : Inport  Port=2
  Abs : Abs  SaturateOnIntegerOverflow=on
  Constant : Constant  Value=w_EG_upper
  Maximum torque : Lookup  InputValues=w_EG_row  Table=T_EG_max  SaturateOnIntegerOverflow=on
  Saturation : Saturate  UpperLimit=0  LowerLimit=-inf
  Saturation1 : Saturate  UpperLimit=0  LowerLimit=-inf
  Stop Simulation : Stop
  Stop Simulation1 : Stop
  Sum : Sum  Inputs=+-  InputSameDT=on  SaturateOnIntegerOverflow=on  OutDataTypeStr=Inherit: Same as first input
  Sum1 : Sum  Inputs=+-  InputSameDT=on  SaturateOnIntegerOverflow=on  OutDataTypeStr=Inherit: Same as first input
  Unit Delay : UnitDelay  SampleTime=-1  HasFrameUpgradeWarning=on
  Unit Delay1 : UnitDelay  SampleTime=-1  HasFrameUpgradeWarning=on
  wires:
  Unit Delay1/1 -> Stop Simulation/1
  Unit Delay/1 -> Stop Simulation1/1
  Saturation1/1 -> Unit Delay/1
  Sum1/1 -> Saturation1/1
  Constant/1 -> Sum1/1
  Saturation/1 -> Unit Delay1/1
  Abs/1 -> Sum/2
  Maximum torque/1 -> Sum/1
  T_EG/1 -> Abs/1
  w_EG/1 -> Sum1/2, Maximum torque/1
  Sum/1 -> Saturation/1

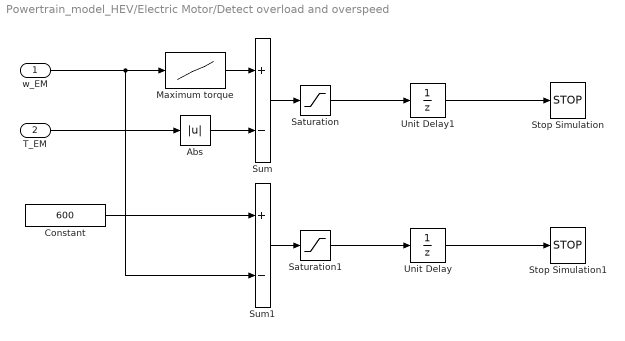
== system Powertrain_model_HEV/Electric Motor/Detect overload and overspeed ==
  w_EM : Inport
  T_EM : Inport  Port=2
  Abs : Abs  SaturateOnIntegerOverflow=on
  Constant : Constant  Value=600
  Maximum torque : Lookup  InputValues=w_EM_row  Table=T_EM_max  SaturateOnIntegerOverflow=on
  Saturation : Saturate  UpperLimit=0  LowerLimit=-inf
  Saturation1 : Saturate  UpperLimit=0  LowerLimit=-inf
  Stop Simulation : Stop
  Stop Simulation1 : Stop
  Sum : Sum  Inputs=+-  InputSameDT=on  SaturateOnIntegerOverflow=on  OutDataTypeStr=Inherit: Same as first input
  Sum1 : Sum  Inputs=+-  InputSameDT=on  SaturateOnIntegerOverflow=on  OutDataTypeStr=Inherit: Same as first input
  Unit Delay : UnitDelay  SampleTime=-1  HasFrameUpgradeWarning=on
  Unit Delay1 : UnitDelay  SampleTime=-1  HasFrameUpgradeWarning=on
  wires:
  Unit Delay1/1 -> Stop Simulation/1
  Unit Delay/1 -> Stop Simulation1/1
  Sum/1 -> Saturation/1
  w_EM/1 -> Maximum torque/1, Sum1/2
  T_EM/1 -> Abs/1
  Maximum torque/1 -> Sum/1
  Abs/1 -> Sum/2
  Saturation/1 -> Unit Delay1/1
  Constant/1 -> Sum1/1
  Sum1/1 -> Saturation1/1
  Saturation1/1 -> Unit Delay/1

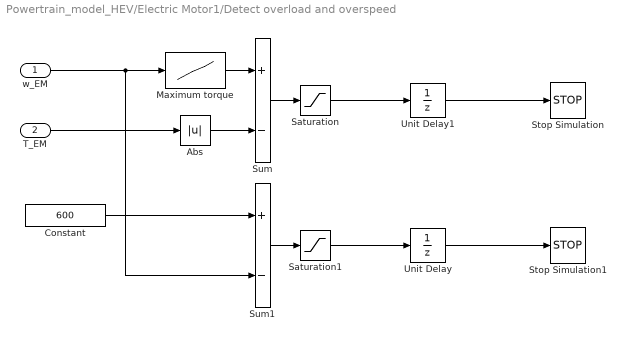
== system Powertrain_model_HEV/Electric Motor1/Detect overload and overspeed ==
  w_EM : Inport
  T_EM : Inport  Port=2
  Abs : Abs  SaturateOnIntegerOverflow=on
  Constant : Constant  Value=600
  Maximum torque : Lookup  InputValues=w_EM_row  Table=T_EM_max  SaturateOnIntegerOverflow=on
  Saturation : Saturate  UpperLimit=0  LowerLimit=-inf
  Saturation1 : Saturate  UpperLimit=0  LowerLimit=-inf
  Stop Simulation : Stop
  Stop Simulation1 : Stop
  Sum : Sum  Inputs=+-  InputSameDT=on  SaturateOnIntegerOverflow=on  OutDataTypeStr=Inherit: Same as first input
  Sum1 : Sum  Inputs=+-  InputSameDT=on  SaturateOnIntegerOverflow=on  OutDataTypeStr=Inherit: Same as first input
  Unit Delay : UnitDelay  SampleTime=-1  HasFrameUpgradeWarning=on
  Unit Delay1 : UnitDelay  SampleTime=-1  HasFrameUpgradeWarning=on
  wires:
  Saturation1/1 -> Unit Delay/1
  Sum1/1 -> Saturation1/1
  Constant/1 -> Sum1/1
  Saturation/1 -> Unit Delay1/1
  Abs/1 -> Sum/2
  Maximum torque/1 -> Sum/1
  T_EM/1 -> Abs/1
  w_EM/1 -> Sum1/2, Maximum torque/1
  Sum/1 -> Saturation/1
  Unit Delay/1 -> Stop Simulation1/1
  Unit Delay1/1 -> Stop Simulation/1

== matlab function Powertrain_model_HEV/Combustion Engine (consumption map)1/MATLAB Function1 ==
  data: rpm input; fuel output; pow input
function fuel   = fuel_con_map(rpm,pow)
x = (rpm-1180)/409.7;
y = (pow-876.1)/438.6;
p00 =         203;
p10 =      0.9394;
p01 =      -8.327;
p20 =       1.894;
p11 =     -0.7168;
p02 =       1.321;
p30 =      0.2621;
p21 =       1.482;
p12 =       5.529;
p03 =      -2.619;
p40 =      0.9252;
p31 =      -3.236;
p22 =       3.413;
p13 =      -2.546;
p04 =        2.97;
p50 =     -0.1717;
p41 =       1.492;
p32 =      -2.908;
p23 =      0.2029;
p14 =      0.4508;
p05 =     -0.7973;
fuel = p00 + p10*x + p01*y + p20*x^2 + p11*x*y + p02*y^2 + p30*x^3 + p21*x^2*y ...
         + p12*x*y^2 + p03*y^3 + p40*x^4 + p31*x^3*y + p22*x^2*y^2 ...
         + p13*x*y^3 + p04*y^4 + p50*x^5 + p41*x^4*y + p32*x^3*y^2 ...
          + p23*x^2*y^3 + p14*x*y^4 + p05*y^5;
end

== matlab function Powertrain_model_HEV/Combustion Engine (consumption map)2/MATLAB Function1 ==
  data: rpm input; fuel output; pow input
function fuel   = fuel_con_map(rpm,pow)
x = (rpm-1180)/409.7;
y = (pow-876.1)/438.6;
p00 =         203;
p10 =      0.9394;
p01 =      -8.327;
p20 =       1.894;
p11 =     -0.7168;
p02 =       1.321;
p30 =      0.2621;
p21 =       1.482;
p12 =       5.529;
p03 =      -2.619;
p40 =      0.9252;
p31 =      -3.236;
p22 =       3.413;
p13 =      -2.546;
p04 =        2.97;
p50 =     -0.1717;
p41 =       1.492;
p32 =      -2.908;
p23 =      0.2029;
p14 =      0.4508;
p05 =     -0.7973;
fuel = p00 + p10*x + p01*y + p20*x^2 + p11*x*y + p02*y^2 + p30*x^3 + p21*x^2*y ...
         + p12*x*y^2 + p03*y^3 + p40*x^4 + p31*x^3*y + p22*x^2*y^2 ...
         + p13*x*y^3 + p04*y^4 + p50*x^5 + p41*x^4*y + p32*x^3*y^2 ...
          + p23*x^2*y^3 + p14*x*y^4 + p05*y^5;
end

== matlab function Powertrain_model_HEV/Combustion Engine (consumption map)/MATLAB Function1 ==
  data: rpm input; fuel output; pow input
function fuel   = fuel_con_map(rpm,pow)
x = (rpm-1180)/409.7;
y = (pow-876.1)/438.6;
p00 =         203;
p10 =      0.9394;
p01 =      -8.327;
p20 =       1.894;
p11 =     -0.7168;
p02 =       1.321;
p30 =      0.2621;
p21 =       1.482;
p12 =       5.529;
p03 =      -2.619;
p40 =      0.9252;
p31 =      -3.236;
p22 =       3.413;
p13 =      -2.546;
p04 =        2.97;
p50 =     -0.1717;
p41 =       1.492;
p32 =      -2.908;
p23 =      0.2029;
p14 =      0.4508;
p05 =     -0.7973;
fuel = p00 + p10*x + p01*y + p20*x^2 + p11*x*y + p02*y^2 + p30*x^3 + p21*x^2*y ...
         + p12*x*y^2 + p03*y^3 + p40*x^4 + p31*x^3*y + p22*x^2*y^2 ...
         + p13*x*y^3 + p04*y^4 + p50*x^5 + p41*x^4*y + p32*x^3*y^2 ...
          + p23*x^2*y^3 + p14*x*y^4 + p05*y^5;
end

== matlab function Powertrain_model_HEV/Combustion Engine (consumption map)4/MATLAB Function1 ==
  data: rpm input; fuel output; pow input
function fuel   = fuel_con_map(rpm,pow)
x = (rpm-1180)/409.7;
y = (pow-876.1)/438.6;
p00 =         203;
p10 =      0.9394;
p01 =      -8.327;
p20 =       1.894;
p11 =     -0.7168;
p02 =       1.321;
p30 =      0.2621;
p21 =       1.482;
p12 =       5.529;
p03 =      -2.619;
p40 =      0.9252;
p31 =      -3.236;
p22 =       3.413;
p13 =      -2.546;
p04 =        2.97;
p50 =     -0.1717;
p41 =       1.492;
p32 =      -2.908;
p23 =      0.2029;
p14 =      0.4508;
p05 =     -0.7973;
fuel = p00 + p10*x + p01*y + p20*x^2 + p11*x*y + p02*y^2 + p30*x^3 + p21*x^2*y ...
         + p12*x*y^2 + p03*y^3 + p40*x^4 + p31*x^3*y + p22*x^2*y^2 ...
         + p13*x*y^3 + p04*y^4 + p50*x^5 + p41*x^4*y + p32*x^3*y^2 ...
          + p23*x^2*y^3 + p14*x*y^4 + p05*y^5;
end
